simulink model "tesd"  (R2012b)
settings: Solver=ode45  StartTime=0.0  StopTime=25000  RelTol=1e-3
undefined symbols (not defined in the file or in its folder): pfb_coeff_gen_calc, sfp
undefined symbols (not defined in the file): SL, transtable
libraries: xbsIndex_r4 x5040, casper_library_misc x112, casper_library_delays x24, xps_library x14, maddogLibrary x4, simulink x2
(part 5 of 49)

== system tesd/dataformatter1 ==
  note: put sync bit
      | at lsb of phase
  note: 32bits
  note: 32bits
  note: 32bits
  note: 32bits
  note: 7bits
  note: 0x55
  note: 16bits
  note: 16bits
  note: 16 bits
  note: 1bit
  note: 8 buts
  note: 0xaaaa
  note: 32 bit timestamp
  note: Now we put data backtogether
      | into 32bit buss
  note: This block extracts mag and phase
      | but truncates both numbers
      | to 16 bit.
  note: WE shrunk the mem to total of 32 bits
      | so we dont use all the bits in
      | header info.
      | all coef data go thru, but gets
      | truncated later...
      | we shoudl truncate here
      | to save resources...
  note: Insert header data before pulse data.
      | We write just pulses to outptu memory.
      | So before pulse, we write magix number of 64k,
      | then write channel number,
      | then output pulse data.
  timestamp32_ : Inport
  channel_ : Inport  Port=2
  data : Inport  Port=3
  is_pulse : Inport  Port=4
  wr_data_sel : Inport  Port=5
  Concat1 : xbsIndex_r4/Concat  num_inputs=4  dbl_ovrd=off  block_type=concat
  Concat2 : xbsIndex_r4/Concat  num_inputs=2  dbl_ovrd=off  block_type=concat
  Concat4 : xbsIndex_r4/Concat  num_inputs=2  dbl_ovrd=off  block_type=concat
  Mux21 : xbsIndex_r4/Mux  inputs=4  en=off  latency=0  precision=Full  arith_type=Unsigned  n_bits=16  bin_pt=14  quantization=Truncate  overflow=Wrap  dbl_ovrd=off  block_type=mux
  TSHi : xbsIndex_r4/Slice  nbits=16  boolean_output=off  mode=Lower Bit Location + Width  bit1=0  base1=MSB of Input  bit0=16  base0=LSB of Input  dbl_ovrd=off  block_type=slice
  TSLow : xbsIndex_r4/Slice  nbits=16  boolean_output=off  mode=Lower Bit Location + Width  bit1=0  base1=MSB of Input  bit0=0  base0=LSB of Input  dbl_ovrd=off  block_type=slice
  c2TruncatePolar16_1 : Subsystem
  lsb8_ : xbsIndex_r4/Slice  nbits=8  boolean_output=off  mode=Lower Bit Location + Width  bit1=0  base1=MSB of Input  bit0=0  base0=LSB of Input  dbl_ovrd=off  block_type=slice
  restofbits_ : xbsIndex_r4/Constant  const=85  gui_display_data_type=Fixed-point  arith_type=Unsigned  n_bits=7  bin_pt=0  preci_type=Single  exp_width=8  frac_width=24  explicit_period=on  period=1  equ=P=C  opselect=C  inp2=PCIN>>17  opr=+  inp1=P  carry=CIN  dbl_ovrd=off  block_type=constant
  ui16_1 : xbsIndex_r4/Constant  const=43690  gui_display_data_type=Fixed-point  arith_type=Unsigned  n_bits=16  bin_pt=0  preci_type=Single  exp_width=8  frac_width=24  explicit_period=on  period=1  equ=P=C  opselect=C  inp2=PCIN>>17  opr=+  inp1=P  carry=CIN  dbl_ovrd=off  block_type=constant
  ui16_10 : xbsIndex_r4/Reinterpret  force_arith_type=on  arith_type=Unsigned  force_bin_pt=on  bin_pt=0  block_type=reinterpret
  ui16_2 : xbsIndex_r4/Reinterpret  force_arith_type=on  arith_type=Unsigned  force_bin_pt=on  bin_pt=0  block_type=reinterpret
  ui32_ : xbsIndex_r4/Constant  const=0  gui_display_data_type=Fixed-point  arith_type=Unsigned  n_bits=32  bin_pt=0  preci_type=Single  exp_width=8  frac_width=24  explicit_period=on  period=1  equ=P=C  opselect=C  inp2=PCIN>>17  opr=+  inp1=P  carry=CIN  dbl_ovrd=off  block_type=constant
  dout : Outport
  wires:
  ui16_10/1 -> Concat4/1
  c2TruncatePolar16_1/1(power) -> ui16_10/1
  c2TruncatePolar16_1/2(phase) -> ui16_2/1
  TSHi/1 -> Concat2/1
  TSLow/1 -> Concat1/2
  restofbits_/1 -> Concat1/1
  ui32_/1 -> Mux21/2
  Concat2/1 -> Mux21/3
  Concat1/1 -> Mux21/4
  channel_/1 -> lsb8_/1
  Concat4/1 -> Mux21/5
  wr_data_sel/1 -> Mux21/1
  lsb8_/1 -> Concat1/4
  ui16_1/1 -> Concat2/2
  is_pulse/1 -> Concat1/3
  timestamp32_/1 -> TSLow/1, TSHi/1
  data/1 -> c2TruncatePolar16_1/1(c)
  Mux21/1 -> dout/1
  ui16_2/1 -> Concat4/2

== system tesd/dataformatter2 ==
  note: put sync bit
      | at lsb of phase
  note: 32bits
  note: 32bits
  note: 32bits
  note: 32bits
  note: 7bits
  note: 0x55
  note: 16bits
  note: 16bits
  note: 16 bits
  note: 1bit
  note: 8 buts
  note: 0xaaaa
  note: 32 bit timestamp
  note: Now we put data backtogether
      | into 32bit buss
  note: This block extracts mag and phase
      | but truncates both numbers
      | to 16 bit.
  note: WE shrunk the mem to total of 32 bits
      | so we dont use all the bits in
      | header info.
      | all coef data go thru, but gets
      | truncated later...
      | we shoudl truncate here
      | to save resources...
  note: Insert header data before pulse data.
      | We write just pulses to outptu memory.
      | So before pulse, we write magix number of 64k,
      | then write channel number,
      | then output pulse data.
  timestamp32_ : Inport
  channel_ : Inport  Port=2
  data : Inport  Port=3
  is_pulse : Inport  Port=4
  wr_data_sel : Inport  Port=5
  Concat1 : xbsIndex_r4/Concat  num_inputs=4  dbl_ovrd=off  block_type=concat
  Concat2 : xbsIndex_r4/Concat  num_inputs=2  dbl_ovrd=off  block_type=concat
  Concat4 : xbsIndex_r4/Concat  num_inputs=2  dbl_ovrd=off  block_type=concat
  Mux21 : xbsIndex_r4/Mux  inputs=4  en=off  latency=0  precision=Full  arith_type=Unsigned  n_bits=16  bin_pt=14  quantization=Truncate  overflow=Wrap  dbl_ovrd=off  block_type=mux
  TSHi : xbsIndex_r4/Slice  nbits=16  boolean_output=off  mode=Lower Bit Location + Width  bit1=0  base1=MSB of Input  bit0=16  base0=LSB of Input  dbl_ovrd=off  block_type=slice
  TSLow : xbsIndex_r4/Slice  nbits=16  boolean_output=off  mode=Lower Bit Location + Width  bit1=0  base1=MSB of Input  bit0=0  base0=LSB of Input  dbl_ovrd=off  block_type=slice
  c2TruncatePolar16_1 : Subsystem
  lsb8_ : xbsIndex_r4/Slice  nbits=8  boolean_output=off  mode=Lower Bit Location + Width  bit1=0  base1=MSB of Input  bit0=0  base0=LSB of Input  dbl_ovrd=off  block_type=slice
  restofbits_ : xbsIndex_r4/Constant  const=85  gui_display_data_type=Fixed-point  arith_type=Unsigned  n_bits=7  bin_pt=0  preci_type=Single  exp_width=8  frac_width=24  explicit_period=on  period=1  equ=P=C  opselect=C  inp2=PCIN>>17  opr=+  inp1=P  carry=CIN  dbl_ovrd=off  block_type=constant
  ui16_1 : xbsIndex_r4/Constant  const=43690  gui_display_data_type=Fixed-point  arith_type=Unsigned  n_bits=16  bin_pt=0  preci_type=Single  exp_width=8  frac_width=24  explicit_period=on  period=1  equ=P=C  opselect=C  inp2=PCIN>>17  opr=+  inp1=P  carry=CIN  dbl_ovrd=off  block_type=constant
  ui16_10 : xbsIndex_r4/Reinterpret  force_arith_type=on  arith_type=Unsigned  force_bin_pt=on  bin_pt=0  block_type=reinterpret
  ui16_2 : xbsIndex_r4/Reinterpret  force_arith_type=on  arith_type=Unsigned  force_bin_pt=on  bin_pt=0  block_type=reinterpret
  ui32_ : xbsIndex_r4/Constant  const=0  gui_display_data_type=Fixed-point  arith_type=Unsigned  n_bits=32  bin_pt=0  preci_type=Single  exp_width=8  frac_width=24  explicit_period=on  period=1  equ=P=C  opselect=C  inp2=PCIN>>17  opr=+  inp1=P  carry=CIN  dbl_ovrd=off  block_type=constant
  dout : Outport
  wires:
  ui16_10/1 -> Concat4/1
  c2TruncatePolar16_1/1(power) -> ui16_10/1
  c2TruncatePolar16_1/2(phase) -> ui16_2/1
  TSHi/1 -> Concat2/1
  TSLow/1 -> Concat1/2
  restofbits_/1 -> Concat1/1
  ui32_/1 -> Mux21/2
  Concat2/1 -> Mux21/3
  Concat1/1 -> Mux21/4
  channel_/1 -> lsb8_/1
  Concat4/1 -> Mux21/5
  wr_data_sel/1 -> Mux21/1
  lsb8_/1 -> Concat1/4
  ui16_1/1 -> Concat2/2
  is_pulse/1 -> Concat1/3
  timestamp32_/1 -> TSLow/1, TSHi/1
  data/1 -> c2TruncatePolar16_1/1(c)
  Mux21/1 -> dout/1
  ui16_2/1 -> Concat4/2

== system tesd/edge_detect ==
  in : Inport
  Delay : xbsIndex_r4/Delay  rst=off  infoeditControl=Selection of Reset will increase slice count due to use of real FFs and instead of SRLs  en=off  latency=1  dbl_ovrd=off  reg_retiming=off  block_type=delay
      settings: xl_area=[0, 0, 0, 0, 0, 0, 0]
  Inverter : xbsIndex_r4/Inverter  en=off  latency=0  dbl_ovrd=off  block_type=inv
      settings: xl_area=[0, 0, 0, 0, 0, 0, 0]
  edge_op : xbsIndex_r4/Logical  logical_function=NOR  inputs=2  en=off  latency=0  precision=Full  arith_type=Unsigned  n_bits=8  bin_pt=2  align_bp=on  dbl_ovrd=off  block_type=logical
      settings: xl_area=[0, 0, 0, 0, 0, 0, 0]
  out : Outport
  wires:
  Inverter/1 -> edge_op/1
  edge_op/1 -> out/1
  in/1 -> Inverter/1, Delay/1
  Delay/1 -> edge_op/2

== system tesd/evtfifordB ==
  out_reg : Inport
  assert_reg : xbsIndex_r4/Assert  assert_type=on  type_source=Explicitly  gui_display_data_type=Fixed-point  arith_type=Unsigned  n_bits=32  bin_pt=0  preci_type=Single  exp_width=8  frac_width=24  assert_rate=off  rate_source=Explicitly  period=1  output_port=on  block_type=assert
  cast_gw : xbsIndex_r4/Convert  gui_display_data_type=Fixed-point  arith_type=Unsigned  n_bits=32  bin_pt=0  float_type=Single  exp_bits=8  fraction_bits=24  quantization=Truncate  overflow=Wrap  en=off  latency=0  dbl_ovrd=off  pipeline=off  block_type=convert
  io_delay : xbsIndex_r4/Delay  rst=off  infoeditControl=Selection of Reset will increase slice count due to use of real FFs and instead of SRLs  en=off  latency=0  dbl_ovrd=off  reg_retiming=on  block_type=delay
  reint1 : xbsIndex_r4/Reinterpret  force_arith_type=on  arith_type=Unsigned  force_bin_pt=on  bin_pt=0  block_type=reinterpret
  tesd_evtfifordB_user_data_in : xbsIndex_r4/Gateway Out  inherit_from_input=off  hdl_port=on  timing_constraint=None  locs_specified=off  LOCs={}  UseAsDAC=off  DACChannel='1'  block_type=gatewayout
  sim_out : Outport
  wires:
  io_delay/1 -> cast_gw/1
  cast_gw/1 -> tesd_evtfifordB_user_data_in/1
  tesd_evtfifordB_user_data_in/1 -> sim_out/1
  out_reg/1 -> assert_reg/1
  assert_reg/1 -> reint1/1
  reint1/1 -> io_delay/1

== system tesd/evtfifowrB ==
  out_reg : Inport
  assert_reg : xbsIndex_r4/Assert  assert_type=on  type_source=Explicitly  gui_display_data_type=Fixed-point  arith_type=Unsigned  n_bits=32  bin_pt=0  preci_type=Single  exp_width=8  frac_width=24  assert_rate=off  rate_source=Explicitly  period=1  output_port=on  block_type=assert
  cast_gw : xbsIndex_r4/Convert  gui_display_data_type=Fixed-point  arith_type=Unsigned  n_bits=32  bin_pt=0  float_type=Single  exp_bits=8  fraction_bits=24  quantization=Truncate  overflow=Wrap  en=off  latency=0  dbl_ovrd=off  pipeline=off  block_type=convert
  io_delay : xbsIndex_r4/Delay  rst=off  infoeditControl=Selection of Reset will increase slice count due to use of real FFs and instead of SRLs  en=off  latency=0  dbl_ovrd=off  reg_retiming=on  block_type=delay
  reint1 : xbsIndex_r4/Reinterpret  force_arith_type=on  arith_type=Unsigned  force_bin_pt=on  bin_pt=0  block_type=reinterpret
  tesd_evtfifowrB_user_data_in : xbsIndex_r4/Gateway Out  inherit_from_input=off  hdl_port=on  timing_constraint=None  locs_specified=off  LOCs={}  UseAsDAC=off  DACChannel='1'  block_type=gatewayout
  sim_out : Outport
  wires:
  io_delay/1 -> cast_gw/1
  cast_gw/1 -> tesd_evtfifowrB_user_data_in/1
  tesd_evtfifowrB_user_data_in/1 -> sim_out/1
  out_reg/1 -> assert_reg/1
  assert_reg/1 -> reint1/1
  reint1/1 -> io_delay/1

== system tesd/extract_sync_enable_1 ==
  note: zero phase term, dbg
  note: array of counters.
      | we can clear them from l;inmux
  note: Assume that data is mag, phase.
      | phase is im part
  dvld_in : Inport
  cmplx_din : Inport  Port=2
  chan : Inport  Port=3
  en : Inport  Port=4
  Delay{,2..4} (4 alike) : xbsIndex_r4/Delay  rst=off  infoeditControl=Selection of Reset will increase slice count due to use of real FFs and instead of SRLs  en=on  latency=2  dbl_ovrd=off  reg_retiming=off  block_type=delay
  Delay5 : xbsIndex_r4/Delay  rst=off  infoeditControl=Selection of Reset will increase slice count due to use of real FFs and instead of SRLs  en=off  latency=2  dbl_ovrd=off  reg_retiming=off  block_type=delay
  cmplx_data : xbsIndex_r4/Slice  nbits=36  boolean_output=off  mode=Lower Bit Location + Width  bit1=0  base1=MSB of Input  bit0=0  base0=LSB of Input  dbl_ovrd=off  block_type=slice
  swtsbits_ : xbsIndex_r4/Slice  nbits=2  boolean_output=off  mode=Upper Bit Location + Width  bit1=0  base1=MSB of Input  bit0=0  base0=LSB of Input  dbl_ovrd=off  block_type=slice
  sync_bit1 : xbsIndex_r4/Slice  nbits=1  boolean_output=on  mode=Upper Bit Location + Width  bit1=-2  base1=MSB of Input  bit0=0  base0=LSB of Input  dbl_ovrd=off  block_type=slice
  dvld_out : Outport
  cmplx_dout : Outport  Port=2
  chanout : Outport  Port=3
  sync_out : Outport  Port=4
  swts : Outport  Port=5
  wires:
  cmplx_data/1 -> Delay3/1
  chan/1 -> Delay/1
  dvld_in/1 -> Delay2/1
  Delay3/1 -> cmplx_dout/1
  en/1 -> [enable]
  [enable] -> Delay3/2, Delay4/2, Delay2/2
  Delay/1 -> chanout/1
  [enable] -> Delay/2
  Delay2/1 -> dvld_out/1
  cmplx_din/1 -> swtsbits_/1, sync_bit1/1, cmplx_data/1
  sync_bit1/1 -> Delay4/1
  Delay4/1 -> sync_out/1
  swtsbits_/1 -> Delay5/1
  Delay5/1 -> swts/1

== system tesd/extract_sync_enable_2 ==
  note: zero phase term, dbg
  note: array of counters.
      | we can clear them from l;inmux
  note: Assume that data is mag, phase.
      | phase is im part
  dvld_in : Inport
  cmplx_din : Inport  Port=2
  chan : Inport  Port=3
  en : Inport  Port=4
  Delay : xbsIndex_r4/Delay  rst=off  infoeditControl=Selection of Reset will increase slice count due to use of real FFs and instead of SRLs  en=on  latency=2  dbl_ovrd=off  reg_retiming=off  block_type=delay
  Delay2 : xbsIndex_r4/Delay  rst=off  infoeditControl=Selection of Reset will increase slice count due to use of real FFs and instead of SRLs  en=on  latency=2  dbl_ovrd=off  reg_retiming=off  block_type=delay
  Delay3 : xbsIndex_r4/Delay  rst=off  infoeditControl=Selection of Reset will increase slice count due to use of real FFs and instead of SRLs  en=on  latency=2  dbl_ovrd=off  reg_retiming=off  block_type=delay
  Delay5 : xbsIndex_r4/Delay  rst=off  infoeditControl=Selection of Reset will increase slice count due to use of real FFs and instead of SRLs  en=off  latency=2  dbl_ovrd=off  reg_retiming=off  block_type=delay
  cmplx_data : xbsIndex_r4/Slice  nbits=36  boolean_output=off  mode=Lower Bit Location + Width  bit1=0  base1=MSB of Input  bit0=0  base0=LSB of Input  dbl_ovrd=off  block_type=slice
  swtsbits_ : xbsIndex_r4/Slice  nbits=2  boolean_output=off  mode=Upper Bit Location + Width  bit1=0  base1=MSB of Input  bit0=0  base0=LSB of Input  dbl_ovrd=off  block_type=slice
  dvld_out : Outport
  cmplx_dout : Outport  Port=2
  chanout : Outport  Port=3
  swts : Outport  Port=4
  wires:
  cmplx_data/1 -> Delay3/1
  chan/1 -> Delay/1
  dvld_in/1 -> Delay2/1
  Delay3/1 -> cmplx_dout/1
  en/1 -> [enable]
  [enable] -> Delay3/2, Delay2/2
  Delay/1 -> chanout/1
  [enable] -> Delay/2
  Delay2/1 -> dvld_out/1
  cmplx_din/1 -> swtsbits_/1, cmplx_data/1
  swtsbits_/1 -> Delay5/1
  Delay5/1 -> swts/1
